simulink model "ss_model"  (R2022b)
settings: Solver=VariableStepAuto  StartTime=0.0  StopTime=10.0  MaxStep=0.01  RelTol=1e-3
values from neighbouring files (symbols this model uses):
  A1 = [0 0   1 0 ... (first row only)    [plant.m]
  A2 = [0   1 ... (first row only)    [plant.m]
  B1 = [0 0 ... (first row only)    [plant.m]
  B2 = [0    0 ... (first row only)    [plant.m]
  C1 = eye(4)    [plant.m]
  C2 = eye(2)    [plant.m]
  D1 = zeros(4, 2)    [plant.m]
  D2 = zeros(2)    [plant.m]
settings Model: Creator=Viktor  LastModifiedBy=Viktor

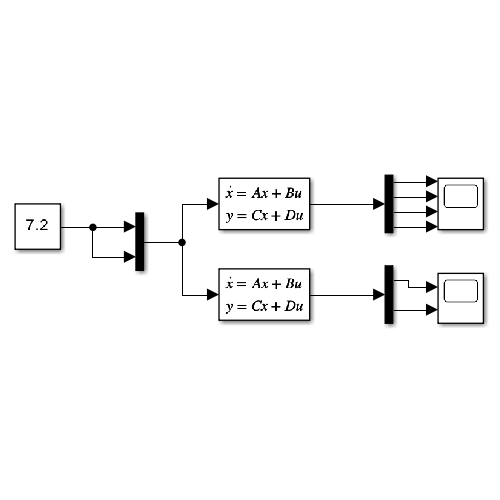
[thumbnail: Simulink's stored preview of the top-level diagram]
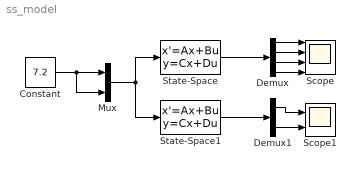
== system ss_model ==
  Constant : Constant  Value=7.2
  Demux : Demux
  Demux1 : Demux  Outputs=2
  Mux : Mux  Inputs=2
  Scope : Scope  NumInputPorts=4
  Scope1 : Scope  NumInputPorts=2
  State-Space : StateSpace  A=A1  B=B1  C=C1  D=D1  InitialCondition=0
  State-Space1 : StateSpace  A=A2  B=B2  C=C2  D=D2  InitialCondition=0
  wires:
  Mux/1 -> State-Space1/1, State-Space/1
  Constant/1 -> Mux/2, Mux/1
  State-Space/1 -> Demux/1
  State-Space1/1 -> Demux1/1
  Demux/1 -> Scope/1
  Demux/2 -> Scope/2
  Demux/3 -> Scope/3
  Demux/4 -> Scope/4
  Demux1/1 -> Scope1/1
  Demux1/2 -> Scope1/2
